simulink model "Speed_Controller_Test_gr"  (Simulink 7.0)
settings: Solver=ode4  SolverMode=SingleTasking  StartTime=0.0  StopTime=252  FixedStep=0.01  RelTol=1e-3
InitFcn:
  | tempomat_para
StopFcn:
  | clear;
values from neighbouring files (symbols this model uses):
  A = 1.9    [tempomat_para.m]
  a_Fzg_max = 2    [tempomat_para.m]
  a_Fzg_min = -2    [tempomat_para.m]
  cw = 0.32    [tempomat_para.m]
  gang = [1 2 3 4]    [tempomat_para.m]
  gang_vec = [1 2 3 4]    [tempomat_para.m]
  i_anteil = 5    [tempomat_para.m]
  i_d = 3.42    [tempomat_para.m]
  i_g = [3.91 2.17 1.37 1.00]    [tempomat_para.m]
  lambda_gang = [1.3 1.25  1.17  1.05]    [tempomat_para.m]
  m_Fzg = 1400    [tempomat_para.m]
  M_mot_max = [130 149 163 170 168 166 162 158 150 139 123 80]    [tempomat_para.m]
  M_mot_min = [0 -40]    [tempomat_para.m]
  n_mot0 = 1000    [tempomat_para.m]
  n_mot_max = 1000:500:6500    [tempomat_para.m]
  n_mot_min = [1000 6500]    [tempomat_para.m]
  p_anteil = 100    [tempomat_para.m]
  r_dyn = 0.28    [tempomat_para.m]
  rho = 1.202    [tempomat_para.m]
  t_sch = 0.2    [tempomat_para.m]
  TI = [block '/TI']    [PSTI_callback.m]
  v_Fzg_ms0 = 0    [tempomat_para.m]
undefined symbols (not defined in the file or in its folder): Drossel_mat, getdatatypespecs
libraries: simulink x116, fzgbib x3
(part 5 of 10)

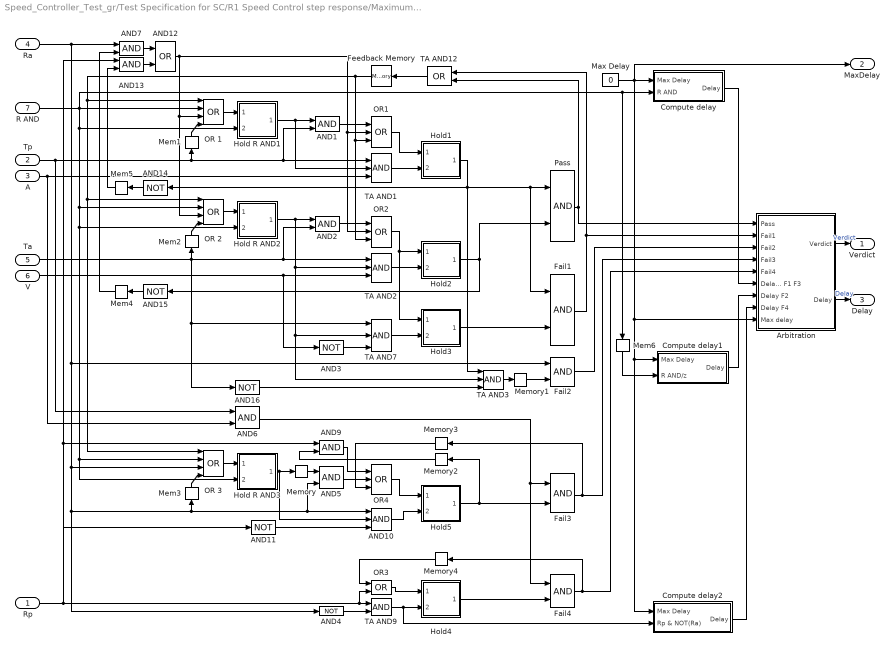
== system Speed_Controller_Test_gr/Test Specification for SC/R1 Speed Control step response/Maximum overshoot < 5 &  Steady state error < 5/PAS1/none - pass - fail ==
  Rp : Inport  OutDataType=sfix(16)  OutScaling=2^0
  Tp : Inport  Port=2  OutDataType=sfix(16)  OutScaling=2^0
  A : Inport  Port=3  OutDataType=sfix(16)  OutScaling=2^0
  Ra : Inport  Port=4  OutDataType=sfix(16)  OutScaling=2^0
  Ta : Inport  Port=5  OutDataType=sfix(16)  OutScaling=2^0
  V : Inport  Port=6  OutDataType=sfix(16)  OutScaling=2^0
  R AND : Inport  Port=7  OutDataType=sfix(16)  OutScaling=2^0
  AND{1..2,5..7,9,13} (7 alike) : Logic  AllPortsSameDT=off  OutDataTypeMode=boolean
  AND10 : Logic  Inputs=3  AllPortsSameDT=off  OutDataTypeMode=boolean
  AND{3..4,11,16} (4 alike) : Logic  Operator=NOT  AllPortsSameDT=off  OutDataTypeMode=boolean
  AND12 : Logic  Operator=OR  AllPortsSameDT=off  OutDataTypeMode=boolean
  AND14 : Logic  Orientation=left  Operator=NOT  AllPortsSameDT=off  OutDataTypeMode=boolean
  AND15 : Logic  Orientation=left  Operator=NOT  AllPortsSameDT=off  OutDataTypeMode=boolean
  Arbitration : Subsystem
  Compute delay : Subsystem
  Compute delay1 : Subsystem
  Compute delay2 : Subsystem
  Fail{1..4} (4 alike) : Logic  AllPortsSameDT=off  OutDataTypeMode=boolean
  Feedback Memory : Memory  Orientation=left
  Hold R AND1 : Subsystem  TreatAsAtomicUnit=on
      mask Display: patch(-0.31+[0.4 0.46 0.46 0.54 0.54 0.6 0.6 0.55 0.55 0.45 0.45 0.4],-0.19+[0.85 0.85 0.95 0.95 0.85 0.85 0.87 0.87 0.96 0.96 0.87 0.87],[0 0 0]);
  Hold R AND2 : Subsystem  TreatAsAtomicUnit=on
      mask Display: patch(-0.31+[0.4 0.46 0.46 0.54 0.54 0.6 0.6 0.55 0.55 0.45 0.45 0.4],-0.19+[0.85 0.85 0.95 0.95 0.85 0.85 0.87 0.87 0.96 0.96 0.87 0.87],[0 0 0]);
  Hold R AND3 : Subsystem  TreatAsAtomicUnit=on
      mask Display: patch(-0.31+[0.4 0.46 0.46 0.54 0.54 0.6 0.6 0.55 0.55 0.45 0.45 0.4],-0.19+[0.85 0.85 0.95 0.95 0.85 0.85 0.87 0.87 0.96 0.96 0.87 0.87],[0 0 0]);
  Hold1 : Subsystem  TreatAsAtomicUnit=on
      mask Display: patch(-0.31+[0.4 0.46 0.46 0.54 0.54 0.6 0.6 0.55 0.55 0.45 0.45 0.4],-0.19+[0.85 0.85 0.95 0.95 0.85 0.85 0.87 0.87 0.96 0.96 0.87 0.87],[0 0 0]);
  Hold2 : Subsystem  TreatAsAtomicUnit=on
      mask Display: patch(-0.31+[0.4 0.46 0.46 0.54 0.54 0.6 0.6 0.55 0.55 0.45 0.45 0.4],-0.19+[0.85 0.85 0.95 0.95 0.85 0.85 0.87 0.87 0.96 0.96 0.87 0.87],[0 0 0]);
  Hold3 : Subsystem  TreatAsAtomicUnit=on
      mask Display: patch(-0.31+[0.4 0.46 0.46 0.54 0.54 0.6 0.6 0.55 0.55 0.45 0.45 0.4],-0.19+[0.85 0.85 0.95 0.95 0.85 0.85 0.87 0.87 0.96 0.96 0.87 0.87],[0 0 0]);
  Hold4 : Subsystem  TreatAsAtomicUnit=on
      mask Display: patch(-0.31+[0.4 0.46 0.46 0.54 0.54 0.6 0.6 0.55 0.55 0.45 0.45 0.4],-0.19+[0.85 0.85 0.95 0.95 0.85 0.85 0.87 0.87 0.96 0.96 0.87 0.87],[0 0 0]);
  Hold5 : Subsystem  TreatAsAtomicUnit=on
      mask Display: patch(-0.31+[0.4 0.46 0.46 0.54 0.54 0.6 0.6 0.55 0.55 0.45 0.45 0.4],-0.19+[0.85 0.85 0.95 0.95 0.85 0.85 0.87 0.87 0.96 0.96 0.87 0.87],[0 0 0]);
  Max Delay : Constant  Value=0  OutDataType=sfix(16)  OutScaling=2^0
  Mem1 : Memory  Orientation=up
  Mem2 : Memory  Orientation=up
  Mem3 : Memory  Orientation=up
  Mem4 : Memory  Orientation=left
  Mem5 : Memory  Orientation=left
  Mem6 : Memory  Orientation=down
  Memory : Memory
  Memory1 : Memory
  Memory2 : Memory  Orientation=left
  Memory3 : Memory  Orientation=left
  Memory4 : Memory  Orientation=left
  OR 1 : Logic  Operator=OR  Inputs=4  AllPortsSameDT=off  OutDataTypeMode=boolean
  OR 2 : Logic  Operator=OR  Inputs=4  AllPortsSameDT=off  OutDataTypeMode=boolean
  OR 3 : Logic  Operator=OR  Inputs=4  AllPortsSameDT=off  OutDataTypeMode=boolean
  OR1 : Logic  Operator=OR  Inputs=3  AllPortsSameDT=off  OutDataTypeMode=boolean
  OR2 : Logic  Operator=OR  Inputs=3  AllPortsSameDT=off  OutDataTypeMode=boolean
  OR3 : Logic  Operator=OR  AllPortsSameDT=off  OutDataTypeMode=boolean
  OR4 : Logic  Operator=OR  Inputs=3  AllPortsSameDT=off  OutDataTypeMode=boolean
  Pass : Logic  AllPortsSameDT=off  OutDataTypeMode=boolean
  TA AND{1..3,7} (4 alike) : Logic  Inputs=3  AllPortsSameDT=off  OutDataTypeMode=boolean
  TA AND12 : Logic  Orientation=left  Operator=OR  AllPortsSameDT=off  OutDataTypeMode=boolean
  TA AND9 : Logic  AllPortsSameDT=off  OutDataTypeMode=boolean
  Verdict : Outport  OutDataType=sfix(16)  OutScaling=2^0
  MaxDelay : Outport  Port=2  OutDataType=sfix(16)  OutScaling=2^0
  Delay : Outport  Port=3  OutDataType=sfix(16)  OutScaling=2^0
  wires:
  Tp/1 -> Mem1/1, TA AND1/1, AND1/2, AND6/1
  OR 1/1 -> Hold R AND1/1(" ")
  A/1 -> TA AND1/3, AND6/2
  Hold1/1("  ") -> Pass/1, Fail1/1, AND14/1, TA AND3/1
  OR1/1 -> Hold1/1(" ")
  TA AND1/1 -> Hold1/2("    ")
  Hold R AND1/1("  ") -> AND1/1, TA AND1/2
  AND1/1 -> OR1/1
  Ta/1 -> Mem2/1, TA AND7/1, AND16/1, AND2/2, TA AND2/1
  OR 2/1 -> Hold R AND2/1(" ")
  V/1 -> AND3/1, TA AND2/3
  Hold2/1("  ") -> AND15/1, Pass/2
  OR2/1 -> Hold2/1(" "), Hold3/1(" ")
  TA AND2/1 -> Hold2/2("    ")
  Hold R AND2/1("  ") -> AND2/1, TA AND3/2, TA AND7/2, TA AND2/2
  AND2/1 -> OR2/1
  Feedback Memory/1 -> OR 1/1, OR 2/1, OR 3/1, OR1/3, OR2/3
  R AND/1 -> OR 2/2, Hold R AND2/2("    "), Hold R AND3/2("    "), OR 3/2, Hold R AND1/2("    "), OR 1/2, Compute delay/2(R AND), Mem6/1
  Ra/1 -> Fail2/1, OR 3/3, AND10/1, AND5/2, Mem3/1, AND4/1, AND7/1
  Mem1/1 -> OR 1/4
  Mem2/1 -> OR 2/4
  TA AND7/1 -> Hold3/2("    ")
  AND3/1 -> TA AND7/3
  TA AND3/1 -> Memory1/1
  Hold3/1("  ") -> Fail1/2
  AND4/1 -> TA AND9/2
  Rp/1 -> AND9/1, AND11/1, AND13/1, TA AND9/1, OR3/2
  TA AND9/1 -> Hold4/2("    "), Compute delay2/2(Rp & NOT(Ra))
  Hold4/1("  ") -> Fail4/2
  OR4/1 -> Hold5/1(" ")
  Hold R AND3/1("  ") -> Memory/1, AND10/2
  OR 3/1 -> Hold R AND3/1(" ")
  Mem3/1 -> OR 3/4
  Memory/1 -> AND5/1
  Hold5/1("  ") -> Memory2/1, Fail3/2
  TA AND12/1 -> Feedback Memory/1
  Fail3/1 -> Memory3/1, Arbitration/4(Fail3)
  Fail4/1 -> Memory4/1, Arbitration/5(Fail4)
  Fail2/1 -> Arbitration/3(Fail2)
  Memory1/1 -> Fail2/2
  AND9/1 -> OR4/1
  Memory2/1 -> AND9/2
  Memory3/1 -> OR4/3
  AND11/1 -> AND10/3
  AND10/1 -> Hold5/2("    ")
  AND5/1 -> OR4/2
  AND7/1 -> AND12/1
  AND13/1 -> AND12/2
  AND12/1 -> OR 1/3, OR 2/3, OR1/2, OR2/2
  Mem4/1 -> AND7/2
  Mem5/1 -> AND13/2
  AND14/1 -> Mem5/1
  AND15/1 -> Mem4/1
  Fail1/1 -> TA AND12/1, Arbitration/2(Fail1)
  AND16/1 -> TA AND3/3
  Pass/1 -> TA AND12/2, Arbitration/1(Pass)
  OR3/1 -> Hold4/1(" ")
  Memory4/1 -> OR3/1
  Max Delay/1 -> Compute delay2/1(Max Delay), Compute delay1/1(Max Delay), Arbitration/9(Max delay), Compute delay/1(Max Delay), MaxDelay/1
  AND6/1 -> Fail3/1, Fail4/1
  Mem6/1 -> Compute delay1/2(R AND/z)
  Compute delay/1(Delay) -> Arbitration/6(Delay P F1 F3)
  Compute delay1/1(Delay) -> Arbitration/7(Delay F2)
  Compute delay2/1(Delay) -> Arbitration/8(Delay F4)
  Arbitration/1(Verdict) -> Verdict/1  "Verdict"
  Arbitration/2(Delay) -> Delay/1  "Delay"

== system Speed_Controller_Test_gr/Test Specification for SC/R1 Speed Control step response/Maximum overshoot < 5 &  Steady state error < 5/Step response characteristics/Step response characteristics extraction ==
  R : Inport  OutDataType=sfix(16)  OutScaling=2^0
  Step : Inport  Port=2  OutDataType=sfix(16)  OutScaling=2^0
  Step response : Inport  Port=3  OutDataType=sfix(16)  OutScaling=2^0
  Clock : Clock
      settings: Decimation=10
  Expected set point and step parameters : Subsystem  TreatAsAtomicUnit=on
  Extract maximum overshoot : Subsystem
  Extract rise time : Subsystem
  Extract settling time : Subsystem
  Extract steady state error : Subsystem
  Memory : Memory
  Static Gain : Constant  OutDataType=sfix(16)  OutScaling=2^0
  Step time : Subsystem  TreatAsAtomicUnit=on
  Rise time : Outport  DataType=double  OutDataType=sfix(16)  OutScaling=2^0
  Maximum overshoot : Outport  Port=2  DataType=double  OutDataType=sfix(16)  OutScaling=2^0
  Settling time : Outport  Port=3  DataType=double  OutDataType=sfix(16)  OutScaling=2^0
  Steady state error : Outport  Port=4  DataType=double  OutDataType=sfix(16)  OutScaling=2^0
  wires:
  Extract rise time/1(Rise time) -> Rise time/1
  Extract maximum overshoot/1(Maximum overshoot) -> Maximum overshoot/1
  Extract settling time/1(Settling time) -> Settling time/1
  Static Gain/1 -> Expected set point and step parameters/3(Static Gain)
  R/1 -> Step time/Trigger, Expected set point and step parameters/Trigger, Extract rise time/2(Reset), Extract maximum overshoot/2(Reset), Extract settling time/3(Reset)
  Step/1 -> Memory/1, Expected set point and step parameters/2(Step)
  Clock/1 -> Step time/1(Clock)
  Memory/1 -> Expected set point and step parameters/1(Step/z)
  Extract steady state error/1(ss error) -> Steady state error/1
  Expected set point and step parameters/2(Set point) -> Extract steady state error/2(Set point), Extract settling time/2(Set point), Extract rise time/3(Set point)
  Step time/1(Time) -> Extract settling time/4(Step time)
  Step response/1 -> Extract steady state error/1(Step response), Extract settling time/1(Step response), Extract maximum overshoot/1(Step response), Extract rise time/1(Step response)
  Expected set point and step parameters/3(Response step size) -> Extract rise time/4(Response step size)
  Expected set point and step parameters/1(Step sign) -> Extract maximum overshoot/3(Step sign)

== system Speed_Controller_Test_gr/Test Specification for SC/R1 Speed Control step response/Maximum overshoot < 5 &  Steady state error < 5/Step response characteristics/Step response reset ==
  Step : Inport  OutDataType=sfix(16)  OutScaling=2^0
  Step response : Inport  Port=2  OutDataType=sfix(16)  OutScaling=2^0
  Active if signals constant for some specified time : Subsystem
  Logical Operator : Logic  AllPortsSameDT=off  OutDataTypeMode=boolean
  Memory : Memory
  Step detection : Subsystem  TreatAsAtomicUnit=on  mask(Feature extraction block){StepSize=10}
      mask prompts: StepSize "Minimum step size"
      mask help: Detect a step in the signal. The minimum step size is defined by the user.
      mask CallbackString:
      | if str2double(get_param(gcb,'StepSize')) <= 0
      |     error(['Minimum step size (' get_param(gcb,'StepSize') ') out of range. Please give a value greater than zero.']);
      | else
      |     set_param([gcb '/Min step size'],'Value',get_param(gcb,'StepSize'));
      | end
  R : Outport  OutDataType=sfix(16)  OutScaling=2^0
  wires:
  Step/1 -> Step detection/1(Signal), Active if signals constant for some specified time/2(Signal 2)
  Active if signals constant for some specified time/1(Constant signals) -> Memory/1
  Memory/1 -> Logical Operator/1
  Step response/1 -> Active if signals constant for some specified time/1(Signal1)
  Step detection/1(Step) -> Logical Operator/2
  Logical Operator/1 -> R/1

== system Speed_Controller_Test_gr/Test Specification for SC/R1 Speed Control step response/Maximum overshoot < 5 &  Steady state error < 5/Step response characteristics/Step response trigger ==
  Steady state error : Inport  OutDataType=sfix(16)  OutScaling=2^0
  Step response : Inport  Port=2  OutDataType=sfix(16)  OutScaling=2^0
  Abs : Abs
  Active if signals constant for some specified time : Subsystem
  Compare To Constant : Subsystem  mask(Compare To Constant){relop=<=, const=5, LogicOutDataTypeMode=uint8, ZeroCross=off}
      mask prompts: relop "Operator:"; const "Constant value:"; LogicOutDataTypeMode "Output data type mode:"; ZeroCross "Enable zero crossing detection"
      mask help: Determine how a signal compares to a constant.
      mask init:
      | blkName = gcb;
      | 
      | if strcmp(get_param(gcbh,'LogicOutDataTypeMode'),'boolean')
      | 	setValue = 'Boolean';
      | else
      | 	setValue = 'Specify via dialog';
      | end
      | 
      | set_param([blkName,'/Compare'],'relop',relop, ...
      | 	'LogicOutDataTypeMode', setValue, 'ZeroCross', ZeroCross);
      | 
      | if length(const) == 1
      |  str = [relop,' ',num2str(double(const))];
      | else
      |   str = [relop,' C'];
      | end
      mask StyleString: popup(==|~=|<|<=|>=|>),edit,popup(uint8|boolean),checkbox
      mask Display: disp(str)
  Data Type Conversion : DataTypeConversion  OutDataType=sfix(16)  OutScaling=2^0
  Data Type Conversion1 : DataTypeConversion  OutDataType=sfix(16)  OutScaling=2^0
  Detect increase : Subsystem  TreatAsAtomicUnit=on
  Logical Operator : Logic  AllPortsSameDT=off  OutDataTypeMode=boolean  LogicDataType=double
  Rise time T : Outport  DataType=double  OutDataType=sfix(16)  OutScaling=2^0
  Overshoot T : Outport  Port=2  DataType=double  OutDataType=sfix(16)  OutScaling=2^0
  Settling time T : Outport  Port=3  DataType=double  OutDataType=sfix(16)  OutScaling=2^0
  Steady state error T : Outport  Port=4  DataType=double  OutDataType=sfix(16)  OutScaling=2^0
  wires:
  Data Type Conversion/1 -> Rise time T/1, Overshoot T/1, Settling time T/1
  Data Type Conversion1/1 -> Steady state error T/1
  Active if signals constant for some specified time/1(Constant signals) -> Detect increase/1(Signal)
  Step response/1 -> Active if signals constant for some specified time/1(Signal1), Active if signals constant for some specified time/2(Signal 2)
  Steady state error/1 -> Abs/1
  Compare To Constant/1(y) -> Logical Operator/1
  Abs/1 -> Compare To Constant/1(u)
  Detect increase/1(Increase) -> Logical Operator/2, Data Type Conversion1/1
  Logical Operator/1 -> Data Type Conversion/1

== system Speed_Controller_Test_gr/Test Specification for SC/R2 Speed Control velocity restoration time after simple  acceleration/deceleration/CC active + no target & Speed Control active & step of V_Des = |1|  with time periods >= 7s/PS/Max Delay A ==
  In1 : Inport  OutDataType=sfix(16)  OutScaling=2^0
  Delay : Constant  Value=0  OutDataType=sfix(16)  OutScaling=2^0
  Integer Delay : S-Function  FunctionName=sfix_udelay  Parameters=samptime,vinit,NumDelays,1,1,0  mask(Integer Delay){vinit=0.0, samptime=-1, NumDelays=15}
      mask prompts: vinit "Initial condition:"; samptime "Sample time:"; NumDelays "Number of delays:"
      mask help: Delay a signal N sample periods.
      mask init:
      | if isempty(NumDelays)
      |    NumDelays = 1;
      | end
      mask Display: fprintf(' %d\nZ   ',-1*(NumDelays))
  Switch : Switch  Criteria=u2 ~= 0
  Out1 : Outport  OutDataType=sfix(16)  OutScaling=2^0
  wires:
  Integer Delay/1 -> Switch/1
  Delay/1 -> Switch/2
  In1/1 -> Integer Delay/1, Switch/3
  Switch/1 -> Out1/1

== system Speed_Controller_Test_gr/Test Specification for SC/R2 Speed Control velocity restoration time after simple  acceleration/deceleration/CC active + no target & Speed Control active & step of V_Des = |1|  with time periods >= 7s/PS/Max Delay R ==
  In1 : Inport  OutDataType=sfix(16)  OutScaling=2^0
  Delay : Constant  Value=0  OutDataType=sfix(16)  OutScaling=2^0
  Integer Delay : S-Function  FunctionName=sfix_udelay  Parameters=samptime,vinit,NumDelays,1,1,0  mask(Integer Delay){vinit=0.0, samptime=-1, NumDelays=15}
      mask prompts: vinit "Initial condition:"; samptime "Sample time:"; NumDelays "Number of delays:"
      mask help: Delay a signal N sample periods.
      mask init:
      | if isempty(NumDelays)
      |    NumDelays = 1;
      | end
      mask Display: fprintf(' %d\nZ   ',-1*(NumDelays))
  Switch : Switch  Criteria=u2 ~= 0
  Out1 : Outport  OutDataType=sfix(16)  OutScaling=2^0
  wires:
  Integer Delay/1 -> Switch/1
  Delay/1 -> Switch/2
  In1/1 -> Integer Delay/1, Switch/3
  Switch/1 -> Out1/1

== system Speed_Controller_Test_gr/Test Specification for SC/R2 Speed Control velocity restoration time after simple  acceleration/deceleration/CC active + no target & Speed Control active & step of V_Des = |1|  with time periods >= 7s/PS/Max Delay T ==
  In1 : Inport  OutDataType=sfix(16)  OutScaling=2^0
  Delay : Constant  Value=0  OutDataType=sfix(16)  OutScaling=2^0
  Integer Delay : S-Function  FunctionName=sfix_udelay  Parameters=samptime,vinit,NumDelays,1,1,0  mask(Integer Delay){vinit=0.0, samptime=-1, NumDelays=15}
      mask prompts: vinit "Initial condition:"; samptime "Sample time:"; NumDelays "Number of delays:"
      mask help: Delay a signal N sample periods.
      mask init:
      | if isempty(NumDelays)
      |    NumDelays = 1;
      | end
      mask Display: fprintf(' %d\nZ   ',-1*(NumDelays))
  Switch : Switch  Criteria=u2 ~= 0
  Out1 : Outport  OutDataType=sfix(16)  OutScaling=2^0
  wires:
  Integer Delay/1 -> Switch/1
  Delay/1 -> Switch/2
  In1/1 -> Integer Delay/1, Switch/3
  Switch/1 -> Out1/1

== system Speed_Controller_Test_gr/Test Specification for SC/R2 Speed Control velocity restoration time after simple  acceleration/deceleration/CC active + no target & Speed Control active & step of V_Des = |1|  with time periods >= 7s/PS/OR - AND ==
  ANDop : Logic  Inputs=1  AllPortsSameDT=off  OutDataTypeMode=boolean
  Default : Constant  OutDataType=sfix(16)  OutScaling=2^0
  ORop : Logic  Operator=OR  Inputs=1  AllPortsSameDT=off  OutDataTypeMode=boolean
  OR : Outport  OutDataType=sfix(16)  OutScaling=2^0
  AND : Outport  Port=2  OutDataType=sfix(16)  OutScaling=2^0
  wires:
  ANDop/1 -> AND/1
  ORop/1 -> OR/1
  Default/1 -> ORop/1, ANDop/1

== system Speed_Controller_Test_gr/Test Specification for SC/R2 Speed Control velocity restoration time after simple  acceleration/deceleration/CC active + no target & Speed Control active & step of V_Des = |1|  with time periods >= 7s/PS/TDD ==
  AND : Logic  AllPortsSameDT=off  OutDataTypeMode=boolean
  One : Constant  OutDataType=sfix(16)  OutScaling=2^0
  A : Outport  OutDataType=sfix(16)  OutScaling=2^0
  T : Outport  Port=2  OutDataType=sfix(16)  OutScaling=2^0
  wires:
  AND/1 -> A/1, T/1
  One/1 -> AND/1, AND/2

== system Speed_Controller_Test_gr/Test Specification for SC/R2 Speed Control velocity restoration time after simple  acceleration/deceleration/CC active + no target & Speed Control active & step of V_Des = |1|  with time periods >= 7s/PS/TI ==
  A1 : Inport  OutDataType=sfix(16)  OutScaling=2^0
  A2 : Inport  Port=2  OutDataType=sfix(16)  OutScaling=2^0
  A3 : Inport  Port=3  OutDataType=sfix(16)  OutScaling=2^0
  AND : Logic  Inputs=3  AllPortsSameDT=off  OutDataTypeMode=boolean
  Delays1 : Subsystem  TreatAsAtomicUnit=on  mask{Delay=0}
      mask prompts: Delay "Delay (in simulation steps) for the input signal:"
      mask init:
      | %set_param([gcb '/Discrete Transfer Fcn'],'Denominator',['[' num2str([1 zeros(1,str2double(get_param(gcb,'Delay')))]) ']']);
      mask CallbackString:
      | Delay = str2double(get_param(gcb,'Delay'));
      | if Delay < 0
      |     set_param(gcb,'Delay','0');
      |     error('Only non-negative delays are possible (causality).');
      |     set_param([gcb '/Delay'],'Value','0');
      | elseif Delay == 0
      |     set_param([gcb '/Delay'],'Value','0');
      | else
      |     set_param([gcb '/Integer Delay'],'NumDelays',num2str(Delay));
      |     set_param([gcb '/Delay'],'Value',num2str(Delay));
      | end
      mask Display: text(0.5,0.5,['z^{ ' num2str((-1)*str2double(get_param(gcb,'Delay'))) '}'],'texmode','on');
  Delays2 : Subsystem  TreatAsAtomicUnit=on  mask{Delay=0}
      mask prompts: Delay "Delay (in simulation steps) for the input signal:"
      mask init:
      | %set_param([gcb '/Discrete Transfer Fcn'],'Denominator',['[' num2str([1 zeros(1,str2double(get_param(gcb,'Delay')))]) ']']);
      mask CallbackString:
      | Delay = str2double(get_param(gcb,'Delay'));
      | if Delay < 0
      |     set_param(gcb,'Delay','0');
      |     error('Only non-negative delays are possible (causality).');
      |     set_param([gcb '/Delay'],'Value','0');
      | elseif Delay == 0
      |     set_param([gcb '/Delay'],'Value','0');
      | else
      |     set_param([gcb '/Integer Delay'],'NumDelays',num2str(Delay));
      |     set_param([gcb '/Delay'],'Value',num2str(Delay));
      | end
      mask Display: text(0.5,0.5,['z^{ ' num2str((-1)*str2double(get_param(gcb,'Delay'))) '}'],'texmode','on');
  Delays3 : Subsystem  TreatAsAtomicUnit=on  mask{Delay=0}
      mask prompts: Delay "Delay (in simulation steps) for the input signal:"
      mask init:
      | %set_param([gcb '/Discrete Transfer Fcn'],'Denominator',['[' num2str([1 zeros(1,str2double(get_param(gcb,'Delay')))]) ']']);
      mask CallbackString:
      | Delay = str2double(get_param(gcb,'Delay'));
      | if Delay < 0
      |     set_param(gcb,'Delay','0');
      |     error('Only non-negative delays are possible (causality).');
      |     set_param([gcb '/Delay'],'Value','0');
      | elseif Delay == 0
      |     set_param([gcb '/Delay'],'Value','0');
      | else
      |     set_param([gcb '/Integer Delay'],'NumDelays',num2str(Delay));
      |     set_param([gcb '/Delay'],'Value',num2str(Delay));
      | end
      mask Display: text(0.5,0.5,['z^{ ' num2str((-1)*str2double(get_param(gcb,'Delay'))) '}'],'texmode','on');
  A : Outport  OutDataType=sfix(16)  OutScaling=2^0
  wires:
  AND/1 -> A/1
  A1/1 -> Delays1/1(In1)
  Delays1/1(Out1) -> AND/1
  A2/1 -> Delays2/1(In1)
  Delays2/1(Out1) -> AND/2
  A3/1 -> Delays3/1(In1)
  Delays3/1(Out1) -> AND/3

== system Speed_Controller_Test_gr/Test Specification for SC/R2 Speed Control velocity restoration time after simple  acceleration/deceleration/CC active + no target & Speed Control active & step of V_Des = |1|  with time periods >= 7s/PS/TID ==
  R OR : Inport  OutDataType=sfix(16)  OutScaling=2^0
  R AND : Inport  Port=2  OutDataType=sfix(16)  OutScaling=2^0
  AND : Logic  Inputs=1  AllPortsSameDT=off  OutDataTypeMode=boolean
  Hold : Subsystem  TreatAsAtomicUnit=on
      mask Display: patch(-0.31+[0.4 0.46 0.46 0.54 0.54 0.6 0.6 0.55 0.55 0.45 0.45 0.4],-0.19+[0.85 0.85 0.95 0.95 0.85 0.85 0.87 0.87 0.96 0.96 0.87 0.87],[0 0 0]);
  A : Outport  OutDataType=sfix(16)  OutScaling=2^0
  T : Outport  Port=2  OutDataType=sfix(16)  OutScaling=2^0
  wires:
  AND/1 -> A/1, T/1
  R AND/1 -> Hold/1(" ")
  R OR/1 -> Hold/2("    ")
  Hold/1("  ") -> AND/1

== system Speed_Controller_Test_gr/Test Specification for SC/R2 Speed Control velocity restoration time after simple  acceleration/deceleration/CC active + no target & Speed Control active & step of V_Des = |1|  with time periods >= 7s/Step with step size=|1|  and time periods >= 6s detection/Step detection ==
  Step : Inport  OutDataType=sfix(16)  OutScaling=2^0
  Active if signals constant for some specified time : Subsystem
  Logical Operator : Logic  AllPortsSameDT=off  OutDataTypeMode=boolean
  Memory : Memory
  Step detection : Subsystem  TreatAsAtomicUnit=on  mask(Feature extraction block){StepSize=1}
      mask prompts: StepSize "Step size"
      mask help: Detect a step in the signal. The minimum step size is defined by the user.
      mask CallbackString:
      | if str2double(get_param(gcb,'StepSize')) <= 0
      |     error(['Step size (' get_param(gcb,'StepSize') ') out of range. Please give a value greater than zero.']);
      | else
      |     set_param([gcb '/Step size'],'Value',get_param(gcb,'StepSize'));
      | end
  R : Outport  OutDataType=sfix(16)  OutScaling=2^0
  wires:
  Step/1 -> Active if signals constant for some specified time/1(Signal 2), Step detection/1(Signal)
  Active if signals constant for some specified time/1(Constant signals) -> Memory/1
  Memory/1 -> Logical Operator/1
  Step detection/1(Step) -> Logical Operator/2
  Logical Operator/1 -> R/1

== system Speed_Controller_Test_gr/Test Specification for SC/R2 Speed Control velocity restoration time after simple  acceleration/deceleration/after (6 seconds)  |V_Des-V_Vhcl <= 1.4|/PAS1/A delay ==
  In1 : Inport  OutDataType=sfix(16)  OutScaling=2^0
  Data Type Conversion : DataTypeConversion  OutDataType=sfix(16)  OutScaling=2^0
  Delay : Constant  Value=600  OutDataType=sfix(16)  OutScaling=2^0
  Integer Delay : S-Function  FunctionName=sfix_udelay  Parameters=samptime,vinit,NumDelays,1,1,0  mask(Integer Delay){vinit=0.0, samptime=-1, NumDelays=600}
      mask prompts: vinit "Initial condition:"; samptime "Sample time:"; NumDelays "Number of delays:"
      mask help: Delay a signal N sample periods.
      mask init:
      | if isempty(NumDelays)
      |    NumDelays = 1;
      | end
      mask Display: fprintf(' %d\nZ   ',-1*(NumDelays))
  Switch : Switch  Criteria=u2 ~= 0
  Out1 : Outport  OutDataType=sfix(16)  OutScaling=2^0
  wires:
  Switch/1 -> Data Type Conversion/1
  In1/1 -> Switch/3, Integer Delay/1
  Delay/1 -> Switch/2
  Integer Delay/1 -> Switch/1
  Data Type Conversion/1 -> Out1/1

== system Speed_Controller_Test_gr/Test Specification for SC/R2 Speed Control velocity restoration time after simple  acceleration/deceleration/after (6 seconds)  |V_Des-V_Vhcl <= 1.4|/PAS1/Delay bus signals ==
  ELLin : Inport  OutDataType=sfix(16)  OutScaling=2^0
  EULin : Inport  Port=2  OutDataType=sfix(16)  OutScaling=2^0
  ADin : Inport  Port=3  OutDataType=sfix(16)  OutScaling=2^0
  AD delay : Subsystem  TreatAsAtomicUnit=on  mask{Delay=0}
      mask prompts: Delay "Delay (in simulation steps) for the input signal:"
      mask init:
      | %set_param([gcb '/Discrete Transfer Fcn'],'Denominator',['[' num2str([1 zeros(1,str2double(get_param(gcb,'Delay')))]) ']']);
      mask CallbackString:
      | Delay = str2double(get_param(gcb,'Delay'));
      | if Delay < 0
      |     set_param(gcb,'Delay','0');
      |     error('Only non-negative delays are possible (causality).');
      |     set_param([gcb '/Delay'],'Value','0');
      | elseif Delay == 0
      |     set_param([gcb '/Delay'],'Value','0');
      | else
      |     set_param([gcb '/Integer Delay'],'NumDelays',num2str(Delay));
      |     set_param([gcb '/Delay'],'Value',num2str(Delay));
      | end
      mask Display: text(0.5,0.5,['z^{ ' num2str((-1)*str2double(get_param(gcb,'Delay'))) '}'],'texmode','on');
  ELL delay : Subsystem  TreatAsAtomicUnit=on  mask{Delay=0}
      mask prompts: Delay "Delay (in simulation steps) for the input signal:"
      mask init:
      | %set_param([gcb '/Discrete Transfer Fcn'],'Denominator',['[' num2str([1 zeros(1,str2double(get_param(gcb,'Delay')))]) ']']);
      mask CallbackString:
      | Delay = str2double(get_param(gcb,'Delay'));
      | if Delay < 0
      |     set_param(gcb,'Delay','0');
      |     error('Only non-negative delays are possible (causality).');
      |     set_param([gcb '/Delay'],'Value','0');
      | elseif Delay == 0
      |     set_param([gcb '/Delay'],'Value','0');
      | else
      |     set_param([gcb '/Integer Delay'],'NumDelays',num2str(Delay));
      |     set_param([gcb '/Delay'],'Value',num2str(Delay));
      | end
      mask Display: text(0.5,0.5,['z^{ ' num2str((-1)*str2double(get_param(gcb,'Delay'))) '}'],'texmode','on');
  EUL delay : Subsystem  TreatAsAtomicUnit=on  mask{Delay=0}
      mask prompts: Delay "Delay (in simulation steps) for the input signal:"
      mask init:
      | %set_param([gcb '/Discrete Transfer Fcn'],'Denominator',['[' num2str([1 zeros(1,str2double(get_param(gcb,'Delay')))]) ']']);
      mask CallbackString:
      | Delay = str2double(get_param(gcb,'Delay'));
      | if Delay < 0
      |     set_param(gcb,'Delay','0');
      |     error('Only non-negative delays are possible (causality).');
      |     set_param([gcb '/Delay'],'Value','0');
      | elseif Delay == 0
      |     set_param([gcb '/Delay'],'Value','0');
      | else
      |     set_param([gcb '/Integer Delay'],'NumDelays',num2str(Delay));
      |     set_param([gcb '/Delay'],'Value',num2str(Delay));
      | end
      mask Display: text(0.5,0.5,['z^{ ' num2str((-1)*str2double(get_param(gcb,'Delay'))) '}'],'texmode','on');
  ELLout : Outport  OutDataType=sfix(16)  OutScaling=2^0
  EULout : Outport  Port=2  OutDataType=sfix(16)  OutScaling=2^0
  ADout : Outport  Port=3  OutDataType=sfix(16)  OutScaling=2^0
  wires:
  AD delay/1(Out1) -> ADout/1
  EUL delay/1(Out1) -> EULout/1
  ELL delay/1(Out1) -> ELLout/1
  ADin/1 -> AD delay/1(In1)
  EULin/1 -> EUL delay/1(In1)
  ELLin/1 -> ELL delay/1(In1)

== system Speed_Controller_Test_gr/Test Specification for SC/R2 Speed Control velocity restoration time after simple  acceleration/deceleration/after (6 seconds)  |V_Des-V_Vhcl <= 1.4|/PAS1/Ra delay ==
  In1 : Inport  OutDataType=sfix(16)  OutScaling=2^0
  Data Type Conversion : DataTypeConversion  OutDataType=sfix(16)  OutScaling=2^0
  Delay : Constant  Value=0  OutDataType=sfix(16)  OutScaling=2^0
  Integer Delay : S-Function  FunctionName=sfix_udelay  Parameters=samptime,vinit,NumDelays,1,1,0  mask(Integer Delay){vinit=0.0, samptime=-1, NumDelays=15}
      mask prompts: vinit "Initial condition:"; samptime "Sample time:"; NumDelays "Number of delays:"
      mask help: Delay a signal N sample periods.
      mask init:
      | if isempty(NumDelays)
      |    NumDelays = 1;
      | end
      mask Display: fprintf(' %d\nZ   ',-1*(NumDelays))
  Switch : Switch  Criteria=u2 ~= 0
  Out1 : Outport  OutDataType=sfix(16)  OutScaling=2^0
  wires:
  Switch/1 -> Data Type Conversion/1
  In1/1 -> Switch/3, Integer Delay/1
  Delay/1 -> Switch/2
  Integer Delay/1 -> Switch/1
  Data Type Conversion/1 -> Out1/1

== system Speed_Controller_Test_gr/Test Specification for SC/R2 Speed Control velocity restoration time after simple  acceleration/deceleration/after (6 seconds)  |V_Des-V_Vhcl <= 1.4|/PAS1/Rp delay ==
  In1 : Inport  OutDataType=sfix(16)  OutScaling=2^0
  Data Type Conversion : DataTypeConversion  OutDataType=sfix(16)  OutScaling=2^0
  Delay : Constant  Value=600  OutDataType=sfix(16)  OutScaling=2^0
  Integer Delay : S-Function  FunctionName=sfix_udelay  Parameters=samptime,vinit,NumDelays,1,1,0  mask(Integer Delay){vinit=0.0, samptime=-1, NumDelays=600}
      mask prompts: vinit "Initial condition:"; samptime "Sample time:"; NumDelays "Number of delays:"
      mask help: Delay a signal N sample periods.
      mask init:
      | if isempty(NumDelays)
      |    NumDelays = 1;
      | end
      mask Display: fprintf(' %d\nZ   ',-1*(NumDelays))
  Switch : Switch  Criteria=u2 ~= 0
  Out1 : Outport  OutDataType=sfix(16)  OutScaling=2^0
  wires:
  Switch/1 -> Data Type Conversion/1
  In1/1 -> Switch/3, Integer Delay/1
  Delay/1 -> Switch/2
  Integer Delay/1 -> Switch/1
  Data Type Conversion/1 -> Out1/1

== system Speed_Controller_Test_gr/Test Specification for SC/R2 Speed Control velocity restoration time after simple  acceleration/deceleration/after (6 seconds)  |V_Des-V_Vhcl <= 1.4|/PAS1/Ta delay ==
  In1 : Inport  OutDataType=sfix(16)  OutScaling=2^0
  Data Type Conversion : DataTypeConversion  OutDataType=sfix(16)  OutScaling=2^0
  Delay : Constant  Value=0  OutDataType=sfix(16)  OutScaling=2^0
  Integer Delay : S-Function  FunctionName=sfix_udelay  Parameters=samptime,vinit,NumDelays,1,1,0  mask(Integer Delay){vinit=0.0, samptime=-1, NumDelays=15}
      mask prompts: vinit "Initial condition:"; samptime "Sample time:"; NumDelays "Number of delays:"
      mask help: Delay a signal N sample periods.
      mask init:
      | if isempty(NumDelays)
      |    NumDelays = 1;
      | end
      mask Display: fprintf(' %d\nZ   ',-1*(NumDelays))
  Switch : Switch  Criteria=u2 ~= 0
  Out1 : Outport  OutDataType=sfix(16)  OutScaling=2^0
  wires:
  Switch/1 -> Data Type Conversion/1
  In1/1 -> Switch/3, Integer Delay/1
  Delay/1 -> Switch/2
  Integer Delay/1 -> Switch/1
  Data Type Conversion/1 -> Out1/1

== system Speed_Controller_Test_gr/Test Specification for SC/R2 Speed Control velocity restoration time after simple  acceleration/deceleration/after (6 seconds)  |V_Des-V_Vhcl <= 1.4|/PAS1/Tp delay ==
  In1 : Inport  OutDataType=sfix(16)  OutScaling=2^0
  Data Type Conversion : DataTypeConversion  OutDataType=sfix(16)  OutScaling=2^0
  Delay : Constant  Value=600  OutDataType=sfix(16)  OutScaling=2^0
  Integer Delay : S-Function  FunctionName=sfix_udelay  Parameters=samptime,vinit,NumDelays,1,1,0  mask(Integer Delay){vinit=0.0, samptime=-1, NumDelays=600}
      mask prompts: vinit "Initial condition:"; samptime "Sample time:"; NumDelays "Number of delays:"
      mask help: Delay a signal N sample periods.
      mask init:
      | if isempty(NumDelays)
      |    NumDelays = 1;
      | end
      mask Display: fprintf(' %d\nZ   ',-1*(NumDelays))
  Switch : Switch  Criteria=u2 ~= 0
  Out1 : Outport  OutDataType=sfix(16)  OutScaling=2^0
  wires:
  Switch/1 -> Data Type Conversion/1
  In1/1 -> Switch/3, Integer Delay/1
  Delay/1 -> Switch/2
  Integer Delay/1 -> Switch/1
  Data Type Conversion/1 -> Out1/1

== system Speed_Controller_Test_gr/Test Specification for SC/R2 Speed Control velocity restoration time after simple  acceleration/deceleration/after (6 seconds)  |V_Des-V_Vhcl <= 1.4|/PAS1/V delay ==
  In1 : Inport  OutDataType=sfix(16)  OutScaling=2^0
  Data Type Conversion : DataTypeConversion  OutDataType=sfix(16)  OutScaling=2^0
  Delay : Constant  Value=0  OutDataType=sfix(16)  OutScaling=2^0
  Integer Delay : S-Function  FunctionName=sfix_udelay  Parameters=samptime,vinit,NumDelays,1,1,0  mask(Integer Delay){vinit=0.0, samptime=-1, NumDelays=15}
      mask prompts: vinit "Initial condition:"; samptime "Sample time:"; NumDelays "Number of delays:"
      mask help: Delay a signal N sample periods.
      mask init:
      | if isempty(NumDelays)
      |    NumDelays = 1;
      | end
      mask Display: fprintf(' %d\nZ   ',-1*(NumDelays))
  Switch : Switch  Criteria=u2 ~= 0
  Out1 : Outport  OutDataType=sfix(16)  OutScaling=2^0
  wires:
  Switch/1 -> Data Type Conversion/1
  In1/1 -> Switch/3, Integer Delay/1
  Delay/1 -> Switch/2
  Integer Delay/1 -> Switch/1
  Data Type Conversion/1 -> Out1/1

== system Speed_Controller_Test_gr/Test Specification for SC/R2 Speed Control velocity restoration time after simple  acceleration/deceleration/after (6 seconds)  |V_Des-V_Vhcl <= 1.4|/PAS1/error ==
  Rp : Inport  OutDataType=sfix(16)  OutScaling=2^0
  Tp : Inport  Port=2  OutDataType=sfix(16)  OutScaling=2^0
  A : Inport  Port=3  OutDataType=sfix(16)  OutScaling=2^0
  Ra : Inport  Port=4  OutDataType=sfix(16)  OutScaling=2^0
  Ta : Inport  Port=5  OutDataType=sfix(16)  OutScaling=2^0
  V : Inport  Port=6  OutDataType=sfix(16)  OutScaling=2^0
  Compare To Constant{,2,4,6,8,10} (6 alike) : simulink/Logic and Bit Operations/Compare To Constant  SystemSampleTime=-1  relop===  const=0  LogicOutDataTypeMode=uint8  ZeroCross=off
  Compare To Constant{1,3,5,7,9,11} (6 alike) : simulink/Logic and Bit Operations/Compare To Constant  SystemSampleTime=-1  relop===  const=1  LogicOutDataTypeMode=uint8  ZeroCross=off
  Logical Operator{,1,3..6} (6 alike) : Logic  Operator=NOR  AllPortsSameDT=off  OutDataTypeMode=boolean
  Logical Operator2 : Logic  Operator=OR  Inputs=6  AllPortsSameDT=off  OutDataTypeMode=boolean
  Verror : Outport  OutDataType=sfix(16)  OutScaling=2^0
  wires:
  Compare To Constant9/1 -> Logical Operator5/2
  Compare To Constant8/1 -> Logical Operator5/1
  Ta/1 -> Compare To Constant8/1, Compare To Constant9/1
  Compare To Constant7/1 -> Logical Operator4/2
  Compare To Constant6/1 -> Logical Operator4/1
  Ra/1 -> Compare To Constant7/1, Compare To Constant6/1
  Tp/1 -> Compare To Constant3/1, Compare To Constant2/1
  Rp/1 -> Compare To Constant1/1, Compare To Constant/1
  Logical Operator2/1 -> Verror/1
  Compare To Constant3/1 -> Logical Operator1/2
  Compare To Constant2/1 -> Logical Operator1/1
  Compare To Constant1/1 -> Logical Operator/2
  Compare To Constant/1 -> Logical Operator/1
  Compare To Constant5/1 -> Logical Operator3/2
  Compare To Constant4/1 -> Logical Operator3/1
  A/1 -> Compare To Constant4/1, Compare To Constant5/1
  Compare To Constant11/1 -> Logical Operator6/2
  Compare To Constant10/1 -> Logical Operator6/1
  V/1 -> Compare To Constant10/1, Compare To Constant11/1
  Logical Operator/1 -> Logical Operator2/1
  Logical Operator1/1 -> Logical Operator2/2
  Logical Operator3/1 -> Logical Operator2/3
  Logical Operator4/1 -> Logical Operator2/4
  Logical Operator5/1 -> Logical Operator2/5
  Logical Operator6/1 -> Logical Operator2/6

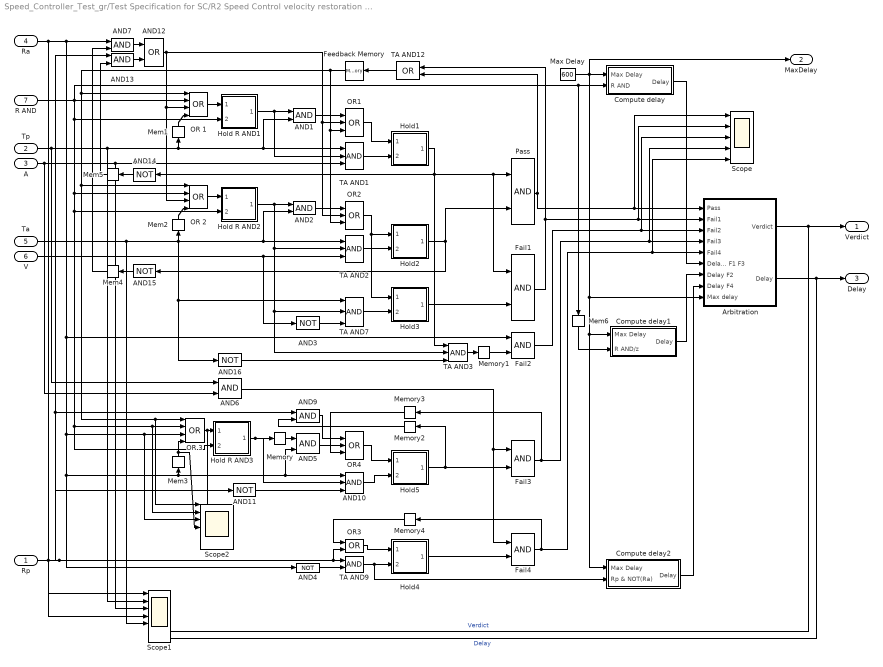
== system Speed_Controller_Test_gr/Test Specification for SC/R2 Speed Control velocity restoration time after simple  acceleration/deceleration/after (6 seconds)  |V_Des-V_Vhcl <= 1.4|/PAS1/none - pass - fail ==
  Rp : Inport  OutDataType=sfix(16)  OutScaling=2^0
  Tp : Inport  Port=2  OutDataType=sfix(16)  OutScaling=2^0
  A : Inport  Port=3  OutDataType=sfix(16)  OutScaling=2^0
  Ra : Inport  Port=4  OutDataType=sfix(16)  OutScaling=2^0
  Ta : Inport  Port=5  OutDataType=sfix(16)  OutScaling=2^0
  V : Inport  Port=6  OutDataType=sfix(16)  OutScaling=2^0
  R AND : Inport  Port=7  OutDataType=sfix(16)  OutScaling=2^0
  AND{1..2,5..7,9,13} (7 alike) : Logic  AllPortsSameDT=off  OutDataTypeMode=boolean
  AND10 : Logic  Inputs=3  AllPortsSameDT=off  OutDataTypeMode=boolean
  AND{3..4,11,16} (4 alike) : Logic  Operator=NOT  AllPortsSameDT=off  OutDataTypeMode=boolean
  AND12 : Logic  Operator=OR  AllPortsSameDT=off  OutDataTypeMode=boolean
  AND14 : Logic  Orientation=left  Operator=NOT  AllPortsSameDT=off  OutDataTypeMode=boolean
  AND15 : Logic  Orientation=left  Operator=NOT  AllPortsSameDT=off  OutDataTypeMode=boolean
  Arbitration : Subsystem
  Compute delay : Subsystem
  Compute delay1 : Subsystem
  Compute delay2 : Subsystem
  Fail{1..4} (4 alike) : Logic  AllPortsSameDT=off  OutDataTypeMode=boolean
  Feedback Memory : Memory  Orientation=left
  Hold R AND1 : Subsystem  TreatAsAtomicUnit=on
      mask Display: patch(-0.31+[0.4 0.46 0.46 0.54 0.54 0.6 0.6 0.55 0.55 0.45 0.45 0.4],-0.19+[0.85 0.85 0.95 0.95 0.85 0.85 0.87 0.87 0.96 0.96 0.87 0.87],[0 0 0]);
  Hold R AND2 : Subsystem  TreatAsAtomicUnit=on
      mask Display: patch(-0.31+[0.4 0.46 0.46 0.54 0.54 0.6 0.6 0.55 0.55 0.45 0.45 0.4],-0.19+[0.85 0.85 0.95 0.95 0.85 0.85 0.87 0.87 0.96 0.96 0.87 0.87],[0 0 0]);
  Hold R AND3 : Subsystem  TreatAsAtomicUnit=on
      mask Display: patch(-0.31+[0.4 0.46 0.46 0.54 0.54 0.6 0.6 0.55 0.55 0.45 0.45 0.4],-0.19+[0.85 0.85 0.95 0.95 0.85 0.85 0.87 0.87 0.96 0.96 0.87 0.87],[0 0 0]);
  Hold1 : Subsystem  TreatAsAtomicUnit=on
      mask Display: patch(-0.31+[0.4 0.46 0.46 0.54 0.54 0.6 0.6 0.55 0.55 0.45 0.45 0.4],-0.19+[0.85 0.85 0.95 0.95 0.85 0.85 0.87 0.87 0.96 0.96 0.87 0.87],[0 0 0]);
  Hold2 : Subsystem  TreatAsAtomicUnit=on
      mask Display: patch(-0.31+[0.4 0.46 0.46 0.54 0.54 0.6 0.6 0.55 0.55 0.45 0.45 0.4],-0.19+[0.85 0.85 0.95 0.95 0.85 0.85 0.87 0.87 0.96 0.96 0.87 0.87],[0 0 0]);
  Hold3 : Subsystem  TreatAsAtomicUnit=on
      mask Display: patch(-0.31+[0.4 0.46 0.46 0.54 0.54 0.6 0.6 0.55 0.55 0.45 0.45 0.4],-0.19+[0.85 0.85 0.95 0.95 0.85 0.85 0.87 0.87 0.96 0.96 0.87 0.87],[0 0 0]);
  Hold4 : Subsystem  TreatAsAtomicUnit=on
      mask Display: patch(-0.31+[0.4 0.46 0.46 0.54 0.54 0.6 0.6 0.55 0.55 0.45 0.45 0.4],-0.19+[0.85 0.85 0.95 0.95 0.85 0.85 0.87 0.87 0.96 0.96 0.87 0.87],[0 0 0]);
  Hold5 : Subsystem  TreatAsAtomicUnit=on
      mask Display: patch(-0.31+[0.4 0.46 0.46 0.54 0.54 0.6 0.6 0.55 0.55 0.45 0.45 0.4],-0.19+[0.85 0.85 0.95 0.95 0.85 0.85 0.87 0.87 0.96 0.96 0.87 0.87],[0 0 0]);
  Max Delay : Constant  Value=600  OutDataType=sfix(16)  OutScaling=2^0
  Mem1 : Memory  Orientation=up
  Mem2 : Memory  Orientation=up
  Mem3 : Memory  Orientation=up
  Mem4 : Memory  Orientation=left
  Mem5 : Memory  Orientation=left
  Mem6 : Memory  Orientation=down
  Memory : Memory
  Memory1 : Memory
  Memory2 : Memory  Orientation=left
  Memory3 : Memory  Orientation=left
  Memory4 : Memory  Orientation=left
  OR 1 : Logic  Operator=OR  Inputs=4  AllPortsSameDT=off  OutDataTypeMode=boolean
  OR 2 : Logic  Operator=OR  Inputs=4  AllPortsSameDT=off  OutDataTypeMode=boolean
  OR 3 : Logic  Operator=OR  Inputs=4  AllPortsSameDT=off  OutDataTypeMode=boolean
  OR1 : Logic  Operator=OR  Inputs=3  AllPortsSameDT=off  OutDataTypeMode=boolean
  OR2 : Logic  Operator=OR  Inputs=3  AllPortsSameDT=off  OutDataTypeMode=boolean
  OR3 : Logic  Operator=OR  AllPortsSameDT=off  OutDataTypeMode=boolean
  OR4 : Logic  Operator=OR  Inputs=3  AllPortsSameDT=off  OutDataTypeMode=boolean
  Pass : Logic  AllPortsSameDT=off  OutDataTypeMode=boolean
  Scope : Scope  NumInputPorts=5
      settings: YMin=-5~-5~-5~-5~-5  YMax=5~5~5~5~5  SaveName=ScopeData9  MaxDataPoints=1115000
  Scope1 : Scope  NumInputPorts=7
      settings: YMin=-5~-5~-5~-5~-5~-5~-5  YMax=5~5~5~5~5~5~5  SaveName=ScopeData10  MaxDataPoints=1115000
  Scope2 : Scope  NumInputPorts=7
      settings: YMin=-5~-5~-5~-5~-5~-5~-5  YMax=5~5~5~5~5~5~5  SaveName=ScopeData11  MaxDataPoints=1115000
  TA AND{1..3,7} (4 alike) : Logic  Inputs=3  AllPortsSameDT=off  OutDataTypeMode=boolean
  TA AND12 : Logic  Orientation=left  Operator=OR  AllPortsSameDT=off  OutDataTypeMode=boolean
  TA AND9 : Logic  AllPortsSameDT=off  OutDataTypeMode=boolean
  Verdict : Outport  OutDataType=sfix(16)  OutScaling=2^0
  MaxDelay : Outport  Port=2  OutDataType=sfix(16)  OutScaling=2^0
  Delay : Outport  Port=3  OutDataType=sfix(16)  OutScaling=2^0
  wires:
  Arbitration/2(Delay) -> Delay/1, Scope1/7  "Delay"
  Arbitration/1(Verdict) -> Verdict/1, Scope1/6  "Verdict"
  Compute delay2/1(Delay) -> Arbitration/8(Delay F4)
  Compute delay1/1(Delay) -> Arbitration/7(Delay F2)
  Compute delay/1(Delay) -> Arbitration/6(Delay P F1 F3)
  Mem6/1 -> Compute delay1/2(R AND/z)
  AND6/1 -> Fail4/1, Fail3/1
  Max Delay/1 -> MaxDelay/1, Compute delay/1(Max Delay), Arbitration/9(Max delay), Compute delay1/1(Max Delay), Compute delay2/1(Max Delay)
  Memory4/1 -> OR3/1
  OR3/1 -> Hold4/1(" ")
  Pass/1 -> TA AND12/2, Arbitration/1(Pass), Scope/1
  AND16/1 -> TA AND3/3
  Fail1/1 -> TA AND12/1, Arbitration/2(Fail1), Scope/2
  AND15/1 -> Mem4/1
  AND14/1 -> Mem5/1
  Mem5/1 -> AND13/2
  Mem4/1 -> AND7/2
  AND12/1 -> OR2/2, OR1/2, OR 2/3, OR 1/3
  AND13/1 -> AND12/2
  AND7/1 -> AND12/1
  AND5/1 -> OR4/2
  AND10/1 -> Hold5/2("    ")
  AND11/1 -> AND10/3
  Memory3/1 -> OR4/3
  Memory2/1 -> AND9/2
  AND9/1 -> OR4/1
  Memory1/1 -> Fail2/2
  Fail2/1 -> Arbitration/3(Fail2), Scope/3
  Fail4/1 -> Memory4/1, Arbitration/5(Fail4), Scope/5
  Fail3/1 -> Memory3/1, Arbitration/4(Fail3), Scope/4
  TA AND12/1 -> Feedback Memory/1
  Hold5/1("  ") -> Fail3/2, Memory2/1
  Mem3/1 -> OR 3/4, Scope2/4
  OR 3/1 -> Hold R AND3/1(" "), Scope2/5
  Hold R AND3/1("  ") -> Memory/1, AND10/2
  OR4/1 -> Hold5/1(" ")
  Hold4/1("  ") -> Fail4/2
  TA AND9/1 -> Compute delay2/2(Rp & NOT(Ra)), Hold4/2("    ")
  Rp/1 -> OR3/2, TA AND9/1, AND13/1, AND11/1, AND9/1, Scope1/1
  AND4/1 -> TA AND9/2
  Hold3/1("  ") -> Fail1/2
  TA AND3/1 -> Memory1/1
  AND3/1 -> TA AND7/3
  TA AND7/1 -> Hold3/2("    ")
  Mem2/1 -> OR 2/4
  Mem1/1 -> OR 1/4
  Ra/1 -> AND7/1, AND4/1, Mem3/1, AND5/2, AND10/1, OR 3/3, Scope2/3, Fail2/1, Scope1/4
  R AND/1 -> Mem6/1, Compute delay/2(R AND), OR 1/2, Hold R AND1/2("    "), Hold R AND3/2("    "), OR 3/2, Scope2/2, Hold R AND2/2("    "), OR 2/2
  Feedback Memory/1 -> OR2/3, OR1/3, OR 2/1, OR 3/1, Scope2/1, OR 1/1
  AND2/1 -> OR2/1
  Hold R AND2/1("  ") -> TA AND2/2, TA AND7/2, TA AND3/2, AND2/1
  TA AND2/1 -> Hold2/2("    ")
  OR2/1 -> Hold3/1(" "), Hold2/1(" ")
  Hold2/1("  ") -> Pass/2, AND15/1
  V/1 -> TA AND2/3, AND3/1
  OR 2/1 -> Hold R AND2/1(" ")
  Ta/1 -> TA AND2/1, AND2/2, AND16/1, TA AND7/1, Mem2/1, Scope1/5
  AND1/1 -> OR1/1
  Hold R AND1/1("  ") -> TA AND1/2, AND1/1
  TA AND1/1 -> Hold1/2("    ")
  OR1/1 -> Hold1/1(" ")
  Hold1/1("  ") -> TA AND3/1, AND14/1, Fail1/1, Pass/1
  A/1 -> AND6/2, TA AND1/3, Scope1/3
  OR 1/1 -> Hold R AND1/1(" ")
  Tp/1 -> AND6/1, AND1/2, TA AND1/1, Mem1/1, Scope1/2
  Memory/1 -> AND5/1

== system Speed_Controller_Test_gr/Test Specification for SC/R2 Speed Control velocity restoration time after simple  acceleration/deceleration/after (6 seconds)  |V_Des-V_Vhcl <= 1.4|/PAS2/A delay ==
  In1 : Inport  OutDataType=sfix(16)  OutScaling=2^0
  Data Type Conversion : DataTypeConversion  OutDataType=sfix(16)  OutScaling=2^0
  Delay : Constant  Value=600  OutDataType=sfix(16)  OutScaling=2^0
  Integer Delay : S-Function  FunctionName=sfix_udelay  Parameters=samptime,vinit,NumDelays,1,1,0  mask(Integer Delay){vinit=0.0, samptime=-1, NumDelays=600}
      mask prompts: vinit "Initial condition:"; samptime "Sample time:"; NumDelays "Number of delays:"
      mask help: Delay a signal N sample periods.
      mask init:
      | if isempty(NumDelays)
      |    NumDelays = 1;
      | end
      mask Display: fprintf(' %d\nZ   ',-1*(NumDelays))
  Switch : Switch  Criteria=u2 ~= 0
  Out1 : Outport  OutDataType=sfix(16)  OutScaling=2^0
  wires:
  Switch/1 -> Data Type Conversion/1
  In1/1 -> Switch/3, Integer Delay/1
  Delay/1 -> Switch/2
  Integer Delay/1 -> Switch/1
  Data Type Conversion/1 -> Out1/1

== system Speed_Controller_Test_gr/Test Specification for SC/R2 Speed Control velocity restoration time after simple  acceleration/deceleration/after (6 seconds)  |V_Des-V_Vhcl <= 1.4|/PAS2/Delay bus signals ==
  ELLin : Inport  OutDataType=sfix(16)  OutScaling=2^0
  EULin : Inport  Port=2  OutDataType=sfix(16)  OutScaling=2^0
  ADin : Inport  Port=3  OutDataType=sfix(16)  OutScaling=2^0
  AD delay : Subsystem  TreatAsAtomicUnit=on  mask{Delay=0}
      mask prompts: Delay "Delay (in simulation steps) for the input signal:"
      mask init:
      | %set_param([gcb '/Discrete Transfer Fcn'],'Denominator',['[' num2str([1 zeros(1,str2double(get_param(gcb,'Delay')))]) ']']);
      mask CallbackString:
      | Delay = str2double(get_param(gcb,'Delay'));
      | if Delay < 0
      |     set_param(gcb,'Delay','0');
      |     error('Only non-negative delays are possible (causality).');
      |     set_param([gcb '/Delay'],'Value','0');
      | elseif Delay == 0
      |     set_param([gcb '/Delay'],'Value','0');
      | else
      |     set_param([gcb '/Integer Delay'],'NumDelays',num2str(Delay));
      |     set_param([gcb '/Delay'],'Value',num2str(Delay));
      | end
      mask Display: text(0.5,0.5,['z^{ ' num2str((-1)*str2double(get_param(gcb,'Delay'))) '}'],'texmode','on');
  ELL delay : Subsystem  TreatAsAtomicUnit=on  mask{Delay=0}
      mask prompts: Delay "Delay (in simulation steps) for the input signal:"
      mask init:
      | %set_param([gcb '/Discrete Transfer Fcn'],'Denominator',['[' num2str([1 zeros(1,str2double(get_param(gcb,'Delay')))]) ']']);
      mask CallbackString:
      | Delay = str2double(get_param(gcb,'Delay'));
      | if Delay < 0
      |     set_param(gcb,'Delay','0');
      |     error('Only non-negative delays are possible (causality).');
      |     set_param([gcb '/Delay'],'Value','0');
      | elseif Delay == 0
      |     set_param([gcb '/Delay'],'Value','0');
      | else
      |     set_param([gcb '/Integer Delay'],'NumDelays',num2str(Delay));
      |     set_param([gcb '/Delay'],'Value',num2str(Delay));
      | end
      mask Display: text(0.5,0.5,['z^{ ' num2str((-1)*str2double(get_param(gcb,'Delay'))) '}'],'texmode','on');
  EUL delay : Subsystem  TreatAsAtomicUnit=on  mask{Delay=0}
      mask prompts: Delay "Delay (in simulation steps) for the input signal:"
      mask init:
      | %set_param([gcb '/Discrete Transfer Fcn'],'Denominator',['[' num2str([1 zeros(1,str2double(get_param(gcb,'Delay')))]) ']']);
      mask CallbackString:
      | Delay = str2double(get_param(gcb,'Delay'));
      | if Delay < 0
      |     set_param(gcb,'Delay','0');
      |     error('Only non-negative delays are possible (causality).');
      |     set_param([gcb '/Delay'],'Value','0');
      | elseif Delay == 0
      |     set_param([gcb '/Delay'],'Value','0');
      | else
      |     set_param([gcb '/Integer Delay'],'NumDelays',num2str(Delay));
      |     set_param([gcb '/Delay'],'Value',num2str(Delay));
      | end
      mask Display: text(0.5,0.5,['z^{ ' num2str((-1)*str2double(get_param(gcb,'Delay'))) '}'],'texmode','on');
  ELLout : Outport  OutDataType=sfix(16)  OutScaling=2^0
  EULout : Outport  Port=2  OutDataType=sfix(16)  OutScaling=2^0
  ADout : Outport  Port=3  OutDataType=sfix(16)  OutScaling=2^0
  wires:
  AD delay/1(Out1) -> ADout/1
  EUL delay/1(Out1) -> EULout/1
  ELL delay/1(Out1) -> ELLout/1
  ADin/1 -> AD delay/1(In1)
  EULin/1 -> EUL delay/1(In1)
  ELLin/1 -> ELL delay/1(In1)
